simulink model "EQ437_24_67AA_709"  (R2024a)
settings: Solver=VariableStepAuto  StartTime=0.0  StopTime=150  RelTol=1e-3
libraries: cstblocks x2
settings Model: Creator=HP  LastModifiedBy=HP

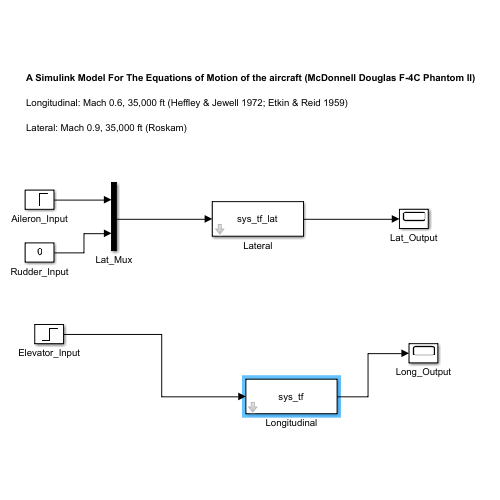
[thumbnail: Simulink's stored preview of the top-level diagram]
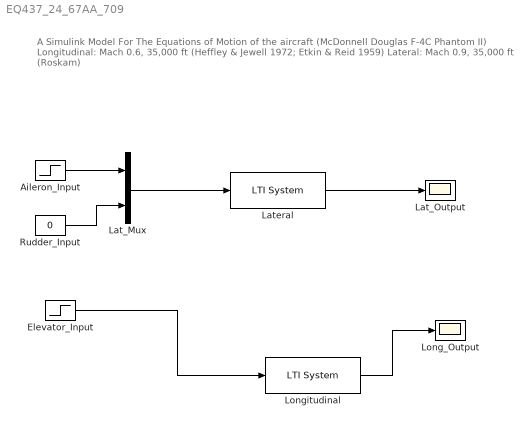
== system EQ437_24_67AA_709 ==
  note: A Simulink Model For The Equations of Motion of the aircraft (McDonnell Douglas F-4C Phantom II)
      |
      | Longitudinal: Mach 0.6, 35,000 ft (Heffley & Jewell 1972; Etkin & Reid 1959)
      |
      | Lateral: Mach 0.9, 35,000 ft (Roskam)
  Aileron_Input : Step  SampleTime=0
  Elevator_Input : Step  SampleTime=0
  Lat_Mux : Mux  Inputs=2
  Lat_Output : Scope
  Lateral : cstblocks/LTI System  sys=sys_tf_lat  IC=[]  PadeOrder=0
  Long_Output : Scope
  Longitudinal : cstblocks/LTI System  sys=sys_tf  IC=[]  PadeOrder=0
  Rudder_Input : Constant  Value=0
  wires:
  Aileron_Input/1 -> Lat_Mux/1
  Lat_Mux/1 -> Lateral/1
  Rudder_Input/1 -> Lat_Mux/2
  Lateral/1 -> Lat_Output/1
  Longitudinal/1 -> Long_Output/1
  Elevator_Input/1 -> Longitudinal/1
